simulink model "vrmanipul"  (Simulink 6.0)
settings: Solver=ode45  StartTime=0.0  StopTime=Inf  RelTol=1e-3
libraries: vrlib x11, simulink x1
settings Model: CovMetricSettings=d  Creator=Houska  LastModifiedBy=Houska  ExtModeTrigMode=oneshot  ExtModeArmWhenConnect=off
settings DataIOCC: SaveOutput=off  SaveTime=off  SignalLoggingName=logsOut
settings OptimizationCC: BlockReduction=off  BooleanDataType=off
settings DebuggingCC: CheckExecutionContextPreStartOutputMsg=on  CheckExecutionContextRuntimeOutputMsg=on  SolverPrmCheckMsg=none
settings HardwareCC: TargetUnknown=on
settings ModelReferenceCC: UpdateModelReferenceTargets=IfOutOfDate
settings GRTTargetCC: LifeSpan=inf
settings SFSimCC: SFSimApplyToAllLibs=on  SFSimBuildMode=Incremental

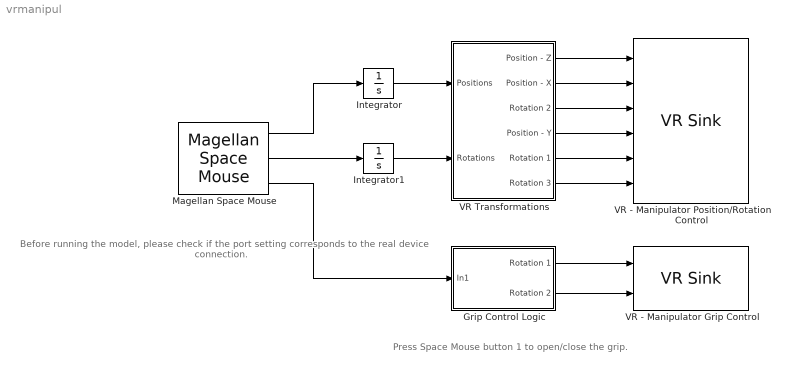
== system vrmanipul ==
  note: Press Space Mouse
      | button 1 to open/close the grip.
  note: Before running the model,
      | please check if the port setting
      | corresponds to the real
      | device connection.
  Grip Control Logic : Subsystem  EnableExecutionContextPropagation=on
  Integrator : Integrator  InitialCondition=[0 -3 0]  LimitOutput=on  UpperSaturationLimit=[4 1 4]  LowerSaturationLimit=[-4 -4 -4]  ZeroCross=off
  Integrator1 : Integrator  InitialCondition=[0 2 0]  UpperSaturationLimit=Inf  LowerSaturationLimit=-Inf  ZeroCross=off
  Magellan Space Mouse : vrlib/Magellan Space Mouse  Port=COM1  OutputType=Speed  Dominant=on  DisableTranslation=off  DisableRotation=off  NormalizeAngle=off  PositionSensitivity=0.001  RotationSensitivity=0.001  InitialPosition=[0 0 0]  InitialRotation=[0 0 0]
  VR - Manipulator Grip Control : vrlib/VR Sink  SampleTime=0  ViewEnable=on  RemoteChange=off  RemoteView=off  FieldsWritten=Finger1.rotation.4#Finger2.rotation.4  WorldFileName=vrmanipul.wrl  WorldDescription=VR Manipulator  AutoView=off  FigureProperties={}
  VR - Manipulator Position/Rotation Control : vrlib/VR Sink  SampleTime=0  ViewEnable=on  RemoteChange=off  RemoteView=off  FieldsWritten=Portal.translation.3.1.double#Base.translation.3.1.double#Telescope.rotation.4.1.double#Telescope.translation.3.1.double#Arm.rotation.4.1.double#Wrist.rotation.4.1.double  WorldFileName=vrmanipul.wrl  AutoView=on
  VR Transformations : Subsystem  EnableExecutionContextPropagation=on
  wires:
  Magellan Space Mouse/3 -> Grip Control Logic/1(In1)
  Magellan Space Mouse/1 -> Integrator/1
  Integrator/1 -> VR Transformations/1(Positions)
  Magellan Space Mouse/2 -> Integrator1/1
  Integrator1/1 -> VR Transformations/2(Rotations)
  VR Transformations/1(Position - Z) -> VR - Manipulator Position/Rotation Control/1
  VR Transformations/2(Position - X) -> VR - Manipulator Position/Rotation Control/2
  VR Transformations/3(Rotation 2) -> VR - Manipulator Position/Rotation Control/3
  VR Transformations/4(Position - Y) -> VR - Manipulator Position/Rotation Control/4
  VR Transformations/5(Rotation 1) -> VR - Manipulator Position/Rotation Control/5
  VR Transformations/6(Rotation 3) -> VR - Manipulator Position/Rotation Control/6
  Grip Control Logic/1(Rotation 1) -> VR - Manipulator Grip Control/1
  Grip Control Logic/2(Rotation 2) -> VR - Manipulator Grip Control/2

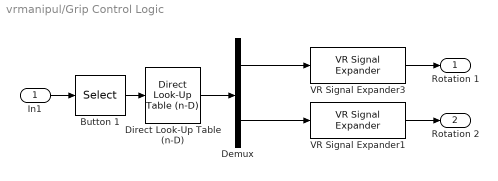
== system vrmanipul/Grip Control Logic ==
  In1 : Inport  LatchInput=off
  Button 1 : Selector
  Demux : Demux  Outputs=2
  Direct Look-Up Table (n-D) : simulink/Look-Up Tables/Direct Look-Up Table (n-D)  maskTabDims=2  explicitNumDims=1  outDims=Column  tabIsInput=off  mxTable=[0.3 0.02;-0.3 -0.02]  clipFlag=Warning
  VR Signal Expander1 : vrlib/VR Signal Expander  outwidth=4  outidx=4
  VR Signal Expander3 : vrlib/VR Signal Expander  outwidth=4  outidx=4
  Rotation 1 : Outport
  Rotation 2 : Outport  Port=2
  wires:
  Button 1/1 -> Direct Look-Up Table (n-D)/1
  Direct Look-Up Table (n-D)/1 -> Demux/1
  Demux/1 -> VR Signal Expander3/1
  Demux/2 -> VR Signal Expander1/1
  VR Signal Expander3/1 -> Rotation 1/1
  In1/1 -> Button 1/1
  VR Signal Expander1/1 -> Rotation 2/1

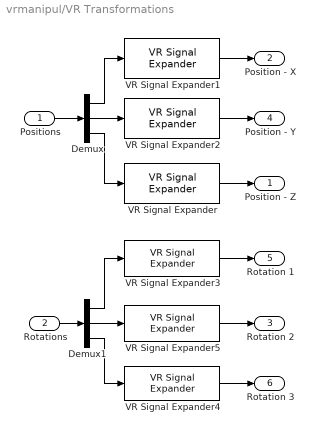
== system vrmanipul/VR Transformations ==
  Positions : Inport  LatchInput=off
  Rotations : Inport  Port=2  LatchInput=off
  Demux : Demux  Outputs=3
  Demux1 : Demux  Outputs=3
  VR Signal Expander : vrlib/VR Signal Expander  outwidth=3  outidx=3
  VR Signal Expander1 : vrlib/VR Signal Expander  outwidth=3  outidx=1
  VR Signal Expander2 : vrlib/VR Signal Expander  outwidth=3  outidx=2
  VR Signal Expander3 : vrlib/VR Signal Expander  outwidth=4  outidx=4
  VR Signal Expander4 : vrlib/VR Signal Expander  outwidth=4  outidx=4
  VR Signal Expander5 : vrlib/VR Signal Expander  outwidth=4  outidx=4
  Position - Z : Outport
  Position - X : Outport  Port=2
  Rotation 2 : Outport  Port=3
  Position - Y : Outport  Port=4
  Rotation 1 : Outport  Port=5
  Rotation 3 : Outport  Port=6
  wires:
  Positions/1 -> Demux/1
  Rotations/1 -> Demux1/1
  VR Signal Expander/1 -> Position - Z/1
  VR Signal Expander1/1 -> Position - X/1
  VR Signal Expander2/1 -> Position - Y/1
  VR Signal Expander3/1 -> Rotation 1/1
  Demux1/1 -> VR Signal Expander3/1
  VR Signal Expander4/1 -> Rotation 3/1
  VR Signal Expander5/1 -> Rotation 2/1
  Demux1/2 -> VR Signal Expander5/1
  Demux1/3 -> VR Signal Expander4/1
  Demux/1 -> VR Signal Expander1/1
  Demux/2 -> VR Signal Expander2/1
  Demux/3 -> VR Signal Expander/1
